simulink model "conversion"  (Simulink 7.0)
settings: Solver=ode45  StartTime=0.0  StopTime=10.0  RelTol=1e-3
settings Model: Creator=root  LastModifiedBy=root  ExtModeAutoUpdateStatusClock=off

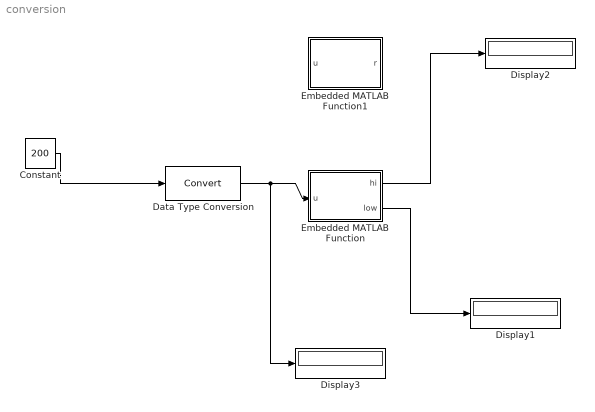
== system conversion ==
  Constant : Constant  Value=200  OutDataType=sfix(16)  OutScaling=2^0
  Data Type Conversion : DataTypeConversion  OutDataTypeMode=uint8  OutDataType=sfix(16)  OutScaling=2^0
  Display1 : Display
  Display2 : Display
  Display3 : Display
  Embedded MATLAB Function : Stateflow chart
  Embedded MATLAB Function1 : Stateflow chart
  wires:
  Constant/1 -> Data Type Conversion/1
  Embedded MATLAB Function/2(low) -> Display1/1
  Embedded MATLAB Function/1(hi) -> Display2/1
  Data Type Conversion/1 -> Embedded MATLAB Function/1(u), Display3/1

== matlab function Embedded MATLAB Function1 ==
  data: u input inherited; r output inherited
function r  = fcn(u)
% This block supports the Embedded MATLAB subset.
% See the help menu for details. 

N=201;

n=N;
i=0;
while n>16
    n=n/16;
% N=floor(a);
i=i+1;
end

r=zeros(1,i+1);

for k=1:i;
N=floor(N/16);
r(i)=rem(N,16);
end

r(i+1)=N;


% 
% 
% [f,e] = log2(double(max(d)));%#ok
% n = max(n,ceil(e/4));
% n0 = n;
% 
% if numD>1
%     n = n*ones(numD,1);
% end
% 
% %For small enough numbers, we can do this the fast way.
% if all(d<bits32),
%     h = sprintf('%0*X',[n,d]');
% else
%     %Division acts differently for integers
%     d = double(d);
%     d1 = floor(d/bits32);
%     d2 = rem(d,bits32);
%     h = sprintf('%0*X%08X',[n-8,d1,d2]');
% end
% 
% h = reshape(h,n0,numD)';

== matlab function Embedded MATLAB Function ==
  data: u input inherited; hi output inherited; low output inherited
function [hi,low] = fcn(u)
% This block supports the Embedded MATLAB subset.
% See the help menu for details. 

a1=u/16;

function h = dec2hex(d,n)
%DEC2HEX Convert decimal integer to hexadecimal string.
%   DEC2HEX(D) returns a 2-D string array where each row is the
%   hexadecimal representation of each decimal integer in D.
%   D must contain non-negative integers smaller than 2^52.
%
%   DEC2HEX(D,N) produces a 2-D string array where each
%   row contains an N digit hexadecimal number.
%
%   Example
%       dec2hex(2748) returns 'ABC'.
%
%   See also HEX2DEC, HEX2NUM, DEC2BIN, DEC2BASE.

%   Copyright 1984-2006 The MathWorks, Inc.
%   $Revision: 5.15.4.7 $  $Date: 2006/11/11 22:45:03 $

bits32 = 4294967296;       % 2^32

if nargin<1
    error(nargchk(1,2,nargin,'struct'));
end

d = d(:); % Make sure d is a column vector.

if ~isreal(d) || any(d < 0) || any(d ~= fix(d))
    error('MATALAB:dec2hex:FirstArgIsInvalid','First argument must contain non-negative integers.')
end
if any(d > 1/eps)
    warning('MATLAB:dec2hex:TooLargeArg',...
        ['At least one of the input numbers is larger than the largest',...
        'FLINT (2^52).\n         Results may be unpredictable.']);
end

numD = numel(d);

if nargin==1,
    n = 1; % Need at least one digit even for 0.
end

[f,e] = log2(double(max(d)));%#ok
n = max(n,ceil(e/4));
n0 = n;

if numD>1
    n = n*ones(numD,1);
end

%For small enough numbers, we can do this the fast way.
if all(d<bits32),
    h = sprintf('%0*X',[n,d]');
else
    %Division acts differently for integers
    d = double(d);
    d1 = floor(d/bits32);
    d2 = rem(d,bits32);
    h = sprintf('%0*X%08X',[n-8,d1,d2]');
end

h = reshape(h,n0,numD)';
